simulink model "Motor_Cmd_varY_expResults"  (Simulink 7.8)
settings: Solver=FixedStepDiscrete  StartTime=0.0  StopTime=10.0  RelTol=1e-3
PreLoadFcn:
  | Motor_Cmd_varY_selfinit
settings Model: SldvGeneratedHarnessModel=TestUnitModel=Motor_Cmd_varY|  Creator=fguerin  LastModifiedBy=klindqvi  CovMetricSettings=dcmoe  CovHTMLOptions=-aTS=1 -bRG=1 -bTC=0 -hTR=0 -nFC=0 -scm=1 -bcm=1  CovModelRefEnable=on  CovExternalEMLEnable=on
settings DataIOCC: LimitDataPoints=off  SaveFormat=StructureWithTime  SaveOutput=off  SignalLogging=off  DSMLogging=off  SaveTime=off  SignalLoggingName=logsOut
settings OptimizationCC: InlineParams=on  InlineInvariantSignals=on  EnhancedBackFolding=on  PassReuseOutputArgsAs=Individual arguments  ZeroExternalMemoryAtStartup=off  ZeroInternalMemoryAtStartup=off  EfficientFloat2IntCast=on  OptimizeModelRefInitCode=on
settings DebuggingCC: SignalInfNanChecking=error  SignalRangeChecking=error  ReadBeforeWriteMsg=EnableAllAsError  WriteAfterWriteMsg=EnableAllAsError  WriteAfterReadMsg=EnableAllAsError  AlgebraicLoopMsg=error  ArtificialAlgebraicLoopMsg=error  SaveWithDisabledLinksMsg=error  SaveWithParameterizedLinksMsg=error  CheckExecutionContextPreStartOutputMsg=on  CheckExecutionContextRuntimeOutputMsg=on  BlockPriorityViolationMsg=error  SolverPrmCheckMsg=error  InheritedTsInSrcMsg=none  MultiTaskCondExecSysMsg=warning  MultiTaskRateTransMsg=warning  CheckMatrixSingularityMsg=error  IntegerOverflowMsg=error  ParameterUnderflowMsg=error  ParameterPrecisionLossMsg=error  ParameterTunabilityLossMsg=error  UnderSpecifiedDataTypeMsg=warning  UnnecessaryDatatypeConvMsg=warning  VectorMatrixConversionMsg=error  SFcnCompatibilityMsg=error  BusObjectLabelMismatch=error  RootOutportRequireBusObject=error  AssertControl=DisableAll  ModelReferenceIOMsg=error  ModelReferenceIOMismatchMessage=error  ModelReferenceCSMismatchMessage=warning  UnknownTsInhSupMsg=error  ModelReferenceDataLoggingMessage=error  StrictBusMsg=ErrorOnBusTreatedAsVector
settings HardwareCC: ProdLargestAtomicInteger=Long  ProdLargestAtomicFloat=Double  ProdIntDivRoundTo=Zero  ProdEndianess=BigEndian  ProdHWDeviceType=Freescale->MPC5500
settings ModelReferenceCC: UpdateModelReferenceTargets=Force
settings SFSimCC: SimParseCustomCode=off
settings RTWCC: SystemTargetFile=autosar.tlc  TemplateMakefile=ert_default_tmf  Description=AUTOSAR  GenerateReport=on  ProcessScript=autosar_make_rtw_hook  IncludeHyperlinkInReport=on  LaunchReport=on  GenerateTraceInfo=on  GenerateTraceReport=on  GenerateTraceReportSl=on  GenerateTraceReportSf=on  GenerateTraceReportEml=on
settings CodeAppCC: ForceParamTrailComments=on  IgnoreCustomStorageClasses=off  IgnoreTestpoints=on  MangleLength=4  InlinedPrmAccess=Macros  ReqsInCode=on
settings STFCustomTargetCC: UtilityFuncGeneration=Shared location  ParMdlRefBuildCompliant=on  CompOptLevelCompliant=on  IncludeMdlTerminateFcn=off  GeneratePreprocessorConditionals=Use local settings  CombineOutputUpdateFcns=on  SuppressErrorStatus=on  ERTFirstTimeCompliant=on  ERTCustomFileBanners=on  SupportAbsoluteTime=off  SupportNonFinite=off  SupportComplex=off  SupportContinuousTime=off  SupportNonInlinedSFcns=off  PortableWordSizes=on  AutosarCompliant=on  SystemTargetFile=autosar.tlc
settings ERTTargetCC: UtilityFuncGeneration=Shared location  MultiwordLength=2048  ConcurrentExecutionCompliant=off  IncludeMdlTerminateFcn=off  SuppressErrorStatus=on  SupportAbsoluteTime=off  SupportNonFinite=off  SupportComplex=off  PortableWordSizes=on  ModelStepFunctionPrototypeControlCompliant=off  CPPClassGenCompliant=off  AutosarCompliant=on  GenerateErtSFunction=on  CreateSILPILBlock=SIL  GenerateASAP2=on  ExtModeMexFile=noextcomm  InlinedParameterPlacement=NonHierarchical  ERTCustomFileTemplate=example_file_process.tlc  ERTFilePackagingFormat=Compact  ConvertIfToSwitch=off  SuppressUnreachableDefaultCases=off
settings CustomProperty: DataType=RTWOptions_EnumType__toolbox_rtw_targets_autosar_autosar_autosar_1_1AutosarSchemaVersion  Value=3.0
settings ConfigComp: Description=Design Verifier Custom Configuration Component  DVMaxProcessTime=600  DVDisplayUnsatisfiableObjectives=on  DVAutomaticStubbing=off  DVOutputDir=C:\Work\Data\Pilots\P_PSA_ECoder_BenchMark_LaGarenne\source9b\deliverable\trunk\demos\VnV_example\Projects\ADL_Project/Simulink_Test_Generation/ADL_Sim  DVModelCoverageObjectives=MCDC  DVTestSuiteOptimization=CombinedObjectives  DVDataFileName=./Tests/$ModelName$_sldvdata  DVSaveHarnessModel=on  DVHarnessModelFileName=./Tests/$ModelName$_testHarness  DVModelReferenceHarness=on  DVSaveReport=on  DVReportFileName=ADL_Sim_SLDV.html

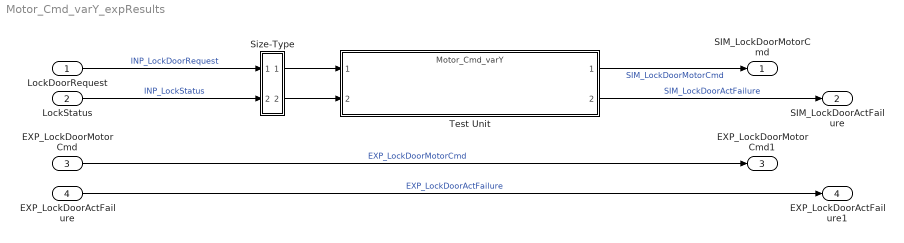
== system Motor_Cmd_varY_expResults ==
  LockDoorRequest : Inport  OutDataTypeStr=boolean  PortDimensions=1
  LockStatus : Inport  Port=2  OutDataTypeStr=Enum: ActuatorStatus  PortDimensions=1
  EXP_LockDoorMotorCmd : Inport  Port=3  OutDataTypeStr=boolean  PortDimensions=1
  EXP_LockDoorActFailure : Inport  Port=4  OutDataTypeStr=Enum: ActuatorStatus  PortDimensions=1
  Size-Type : Subsystem
  Test Unit : ModelReference  ModelNameDialog=Motor_Cmd_varY  SimulationMode=Normal  ModelReferenceVersion=1.41  CopyOfModelName=Motor_Cmd_varY  DefaultDataLogging=off
  SIM_LockDoorMotorCmd : Outport  OutDataTypeStr=uint8  PortDimensions=1
  SIM_LockDoorActFailure : Outport  Port=2  OutDataTypeStr=boolean
  EXP_LockDoorMotorCmd1 : Outport  Port=3  PortDimensions=1
  EXP_LockDoorActFailure1 : Outport  Port=4
  wires:
  LockDoorRequest/1 -> Size-Type/1(In1)  "INP_LockDoorRequest"
  Size-Type/1(Out1) -> Test Unit/1
  LockStatus/1 -> Size-Type/2(In2)  "INP_LockStatus"
  Size-Type/2(Out2) -> Test Unit/2
  Test Unit/1 -> SIM_LockDoorMotorCmd/1  "SIM_LockDoorMotorCmd"
  Test Unit/2 -> SIM_LockDoorActFailure/1  "SIM_LockDoorActFailure"
  EXP_LockDoorMotorCmd/1 -> EXP_LockDoorMotorCmd1/1  "EXP_LockDoorMotorCmd"
  EXP_LockDoorActFailure/1 -> EXP_LockDoorActFailure1/1  "EXP_LockDoorActFailure"

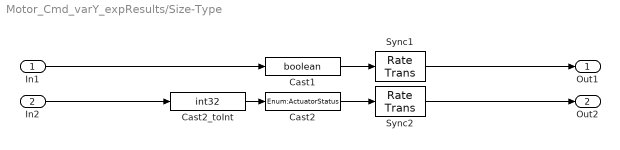
== system Motor_Cmd_varY_expResults/Size-Type ==
  In1 : Inport
  In2 : Inport  Port=2
  Cast1 : DataTypeConversion  OutDataTypeStr=boolean  SaturateOnIntegerOverflow=on  RndMeth=Zero
  Cast2 : DataTypeConversion  OutDataTypeStr=Enum:ActuatorStatus  SaturateOnIntegerOverflow=on  RndMeth=Zero
  Cast2_toInt : DataTypeConversion  OutDataTypeStr=int32  SaturateOnIntegerOverflow=on  RndMeth=Zero
  Sync1 : RateTransition  OutPortSampleTime=[0.20000000000000001,0]
  Sync2 : RateTransition  OutPortSampleTime=[0.20000000000000001,0]
  Out1 : Outport
  Out2 : Outport  Port=2
  wires:
  In1/1 -> Cast1/1
  Cast1/1 -> Sync1/1
  Sync1/1 -> Out1/1
  In2/1 -> Cast2_toInt/1
  Cast2_toInt/1 -> Cast2/1
  Cast2/1 -> Sync2/1
  Sync2/1 -> Out2/1
